simulink model "simRouteA_v4_11"  (R2015a)
settings: Solver=FixedStepDiscrete  StartTime=0.0  StopTime=36000  FixedStep=1  RelTol=1e-3
PreLoadFcn:
  | loadTimetable
StopFcn:
  | postProcess
undefined symbols (not defined in the file or in its folder): setBus1IntergenTime, setBus2IntergenTime, setBus3IntergenTime, setBus4IntergenTime
(part 5 of 7)

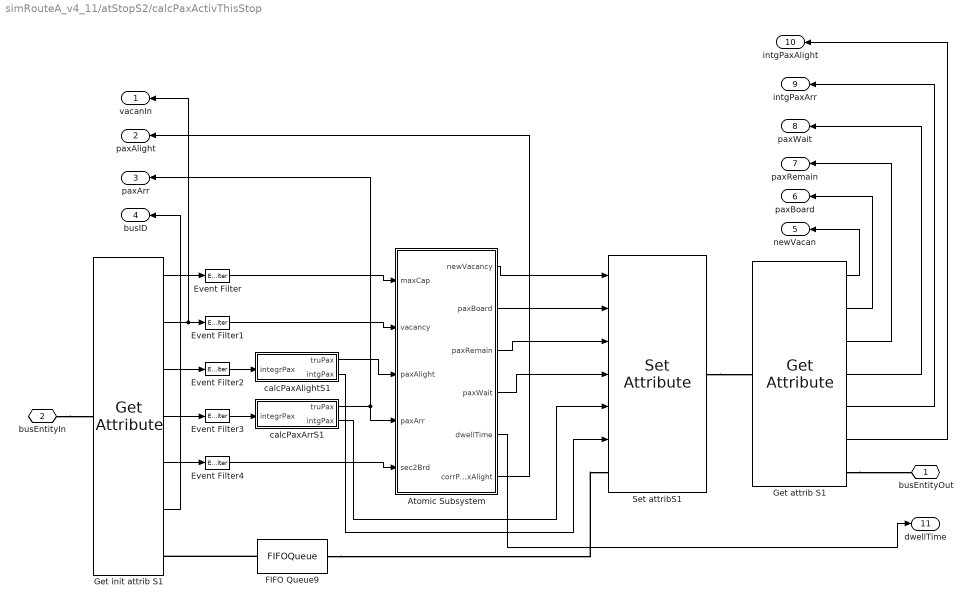
== system simRouteA_v4_11/atStopS2/calcPaxActivThisStop ==
  Atomic Subsystem : Subsystem  TreatAsAtomicUnit=on
  Event Filter{,1..4} (5 alike) : EventFilter  ExecuteSubsystem=Upon sample time hit  SignalEdgeType=Rising
  FIFO Queue9 : FIFOQueue
  Get attrib S1 : GetAttribute  AttributeName=vacancy|paxBoard|paxRemain|paxWait|intgPaxArr|intgPaxAlight  AttributeMissing=Error|Error|Error|Error|Error|Error  AttributeDefaultValue=1|1|1|1|1|1  AttributeTreatAsVector=1|1|1|1|1|1  AttributeSendTiming=After entity departure|After entity departure|After entity departure|After entity departure|After entity departure|After entity departure  EvaluatedDefaultAttributeValue={ []; []; []; []; []; []}
      settings: OutputPortMap=o1,o2,o3,o4,o5,o6
  Get init attrib S1 : GetAttribute  AttributeName=maxCap|vacancy|paxAlight|paxArr|sec2Brd|ID  AttributeMissing=Error|Error|Error|Error|Error|Error  AttributeDefaultValue=1|1|1|1|1|1  AttributeTreatAsVector=1|1|1|1|1|1  AttributeSendTiming=After entity departure|After entity departure|After entity departure|After entity departure|After entity departure|After entity departure  EvaluatedDefaultAttributeValue={ []; []; []; []; []; []}
      settings: OutputPortMap=o1,o2,o3,o4,o5,o6
  Set attribS1 : SetAttribute  AttributeName=vacancy|paxBoard|paxRemain|paxWait|intgPaxArr|intgPaxAlight  AttributeFrom=Signal port|Signal port|Signal port|Signal port|Signal port|Signal port  AttributeValue=1|1|1|1|1|1  AttributeTreatAsVector=1|1|1|1|1|1  EvaluatedAttributeValue={ []; []; []; []; []; [] }
      settings: InputPortMap=u0,u1,u2,u3,u4,u5
  calcPaxAlightS1 : Subsystem  TreatAsAtomicUnit=on
  calcPaxArrS1 : Subsystem  TreatAsAtomicUnit=on
  busEntityOut : PMIOPort  Port=1  Side=Right
  busEntityIn : PMIOPort  Port=2  Side=Left
  vacanIn : Outport
  paxAlight : Outport  Port=2
  paxArr : Outport  Port=3
  busID : Outport  Port=4
  newVacan : Outport  Port=5
  paxBoard : Outport  Port=6
  paxRemain : Outport  Port=7
  paxWait : Outport  Port=8
  intgPaxArr : Outport  Port=9
  intgPaxAlight : Outport  Port=10
  dwellTime : Outport  Port=11
  wires:
  Event Filter3/1 -> calcPaxArrS1/1(integrPax)
  Event Filter2/1 -> calcPaxAlightS1/1(integrPax)
  Get init attrib S1/6 -> busID/1
  Get init attrib S1/2 -> vacanIn/1, Event Filter1/1
  Get attrib S1/2 -> paxBoard/1
  Atomic Subsystem/1(newVacancy) -> Set attribS1/1
  Get attrib S1/1 -> newVacan/1
  Get attrib S1/3 -> paxRemain/1
  Get attrib S1/4 -> paxWait/1
  Event Filter/1 -> Atomic Subsystem/1(maxCap)
  Get init attrib S1/5 -> Event Filter4/1
  Atomic Subsystem/5(dwellTime) -> dwellTime/1
  Event Filter1/1 -> Atomic Subsystem/2(vacancy)
  Get init attrib S1/1 -> Event Filter/1
  Event Filter4/1 -> Atomic Subsystem/5(sec2Brd)
  Atomic Subsystem/2(paxBoard) -> Set attribS1/2
  Atomic Subsystem/3(paxRemain) -> Set attribS1/3
  Atomic Subsystem/4(paxWait) -> Set attribS1/4
  Get init attrib S1/4 -> Event Filter3/1
  Get init attrib S1/3 -> Event Filter2/1
  calcPaxAlightS1/1(truPax) -> Atomic Subsystem/3(paxAlight)
  calcPaxArrS1/1(truPax) -> Atomic Subsystem/4(paxArr), paxArr/1
  calcPaxArrS1/2(intgPax) -> Set attribS1/5
  calcPaxAlightS1/2(intgPax) -> Set attribS1/6
  Get attrib S1/5 -> intgPaxArr/1
  Get attrib S1/6 -> intgPaxAlight/1
  Atomic Subsystem/6(corrPaxAlight) -> paxAlight/1
  connections:
  busEntityIn/RConn1 -- Get init attrib S1/LConn1
  FIFO Queue9/LConn1 -- Get init attrib S1/RConn1
  Set attribS1/RConn1 -- Get attrib S1/LConn1
  Get attrib S1/RConn1 -- busEntityOut/RConn1
  FIFO Queue9/RConn1 -- Set attribS1/LConn1

== system simRouteA_v4_11/atStopS2/integrPaxAlightS1 ==
  ratePax : Inport
  Atomic Subsystem1 : Subsystem  TreatAsAtomicUnit=on
  Round1 : Rounding  Operator=round
  T2E1 : TimedToEventSignal
  accPax : Outport
  wires:
  Round1/1 -> T2E1/1
  T2E1/1 -> Atomic Subsystem1/1(In1)
  ratePax/1 -> Round1/1
  Atomic Subsystem1/1(Out1) -> accPax/1

== system simRouteA_v4_11/atStopS2/integrPaxArrS1 ==
  ratePax : Inport
  Atomic Subsystem1 : Subsystem  TreatAsAtomicUnit=on
  Round1 : Rounding  Operator=round
  T2E1 : TimedToEventSignal
  accPax : Outport
  wires:
  Round1/1 -> T2E1/1
  T2E1/1 -> Atomic Subsystem1/1(In1)
  ratePax/1 -> Round1/1
  Atomic Subsystem1/1(Out1) -> accPax/1

== system simRouteA_v4_11/atStopS3/busDwellThisStop ==
  dwellTime : Inport
  Clock2 : Clock
  DummyServer : SingleServer  ServiceTime=0
  FIFO Queue3 : FIFOQueue
  Get Attribute5 : GetAttribute  AttributeName=dwellTime|tStartSrvPax  AttributeMissing=Error|Error  AttributeDefaultValue=1|1  AttributeTreatAsVector=1|1  AttributeSendTiming=After entity departure|After entity departure  EvaluatedDefaultAttributeValue={ []; []}
      settings: OutputPortMap=o1,o2
  Infinite Server : InfiniteServer  ServiceTimeFrom=Signal port t
  Set Attribute3 : SetAttribute  AttributeName=dwellTime|tStartSrvPax  AttributeFrom=Signal port|Signal port  AttributeValue=1|1  AttributeTreatAsVector=1|1  EvaluatedAttributeValue={ []; [] }
      settings: InputPortMap=u0,u1
  Subsystem2 : Subsystem  TreatAsAtomicUnit=on
  T2E4 : TimedToEventSignal
  busWaitAtStop : SingleServer  Commented=on  ServiceTimeFrom=Signal port t
  busesQueueAtStop : FIFOQueue
  getIDBusLeave : GetAttribute  AttributeName=ID  EvaluatedDefaultAttributeValue={ []}
      settings: OutputPortMap=o1
  busOut : PMIOPort  Port=1  Side=Right
  busIn : PMIOPort  Port=2  Side=Left
  idBusLeave : Outport
  wires:
  getIDBusLeave/1 -> idBusLeave/1
  dwellTime/1 -> Set Attribute3/1
  Clock2/1 -> T2E4/1
  T2E4/1 -> Set Attribute3/2
  Get Attribute5/2 -> Subsystem2/2(tStartSrvPax)
  Get Attribute5/1 -> Subsystem2/1(dwellTime)
  Subsystem2/1(dwellTimeNew) -> Infinite Server/1
  connections:
  busIn/RConn1 -- busesQueueAtStop/LConn1
  getIDBusLeave/RConn1 -- busOut/RConn1
  busesQueueAtStop/RConn1 -- Set Attribute3/LConn1
  Infinite Server/RConn1 -- getIDBusLeave/LConn1
  Set Attribute3/RConn1 -- FIFO Queue3/LConn1
  FIFO Queue3/RConn1 -- Get Attribute5/LConn1
  Get Attribute5/RConn1 -- DummyServer/LConn1
  Infinite Server/LConn1 -- DummyServer/RConn1

== system simRouteA_v4_11/atStopS3/calcPaxActivThisStop ==
  Atomic Subsystem : Subsystem  TreatAsAtomicUnit=on
  Event Filter{,1..4} (5 alike) : EventFilter  ExecuteSubsystem=Upon sample time hit  SignalEdgeType=Rising
  FIFO Queue9 : FIFOQueue
  Get attrib S1 : GetAttribute  AttributeName=vacancy|paxBoard|paxRemain|paxWait|intgPaxArr|intgPaxAlight  AttributeMissing=Error|Error|Error|Error|Error|Error  AttributeDefaultValue=1|1|1|1|1|1  AttributeTreatAsVector=1|1|1|1|1|1  AttributeSendTiming=After entity departure|After entity departure|After entity departure|After entity departure|After entity departure|After entity departure  EvaluatedDefaultAttributeValue={ []; []; []; []; []; []}
      settings: OutputPortMap=o1,o2,o3,o4,o5,o6
  Get init attrib S1 : GetAttribute  AttributeName=maxCap|vacancy|paxAlight|paxArr|sec2Brd|ID  AttributeMissing=Error|Error|Error|Error|Error|Error  AttributeDefaultValue=1|1|1|1|1|1  AttributeTreatAsVector=1|1|1|1|1|1  AttributeSendTiming=After entity departure|After entity departure|After entity departure|After entity departure|After entity departure|After entity departure  EvaluatedDefaultAttributeValue={ []; []; []; []; []; []}
      settings: OutputPortMap=o1,o2,o3,o4,o5,o6
  Set attribS1 : SetAttribute  AttributeName=vacancy|paxBoard|paxRemain|paxWait|intgPaxArr|intgPaxAlight  AttributeFrom=Signal port|Signal port|Signal port|Signal port|Signal port|Signal port  AttributeValue=1|1|1|1|1|1  AttributeTreatAsVector=1|1|1|1|1|1  EvaluatedAttributeValue={ []; []; []; []; []; [] }
      settings: InputPortMap=u0,u1,u2,u3,u4,u5
  calcPaxAlightS1 : Subsystem  TreatAsAtomicUnit=on
  calcPaxArrS1 : Subsystem  TreatAsAtomicUnit=on
  busEntityOut : PMIOPort  Port=1  Side=Right
  busEntityIn : PMIOPort  Port=2  Side=Left
  vacanIn : Outport
  paxAlight : Outport  Port=2
  paxArr : Outport  Port=3
  busID : Outport  Port=4
  newVacan : Outport  Port=5
  paxBoard : Outport  Port=6
  paxRemain : Outport  Port=7
  paxWait : Outport  Port=8
  intgPaxArr : Outport  Port=9
  intgPaxAlight : Outport  Port=10
  dwellTime : Outport  Port=11
  wires:
  Event Filter3/1 -> calcPaxArrS1/1(integrPax)
  Event Filter2/1 -> calcPaxAlightS1/1(integrPax)
  Get init attrib S1/6 -> busID/1
  Get init attrib S1/2 -> vacanIn/1, Event Filter1/1
  Get attrib S1/2 -> paxBoard/1
  Atomic Subsystem/1(newVacancy) -> Set attribS1/1
  Get attrib S1/1 -> newVacan/1
  Get attrib S1/3 -> paxRemain/1
  Get attrib S1/4 -> paxWait/1
  Event Filter/1 -> Atomic Subsystem/1(maxCap)
  Get init attrib S1/5 -> Event Filter4/1
  Atomic Subsystem/5(dwellTime) -> dwellTime/1
  Event Filter1/1 -> Atomic Subsystem/2(vacancy)
  Get init attrib S1/1 -> Event Filter/1
  Event Filter4/1 -> Atomic Subsystem/5(sec2Brd)
  Atomic Subsystem/2(paxBoard) -> Set attribS1/2
  Atomic Subsystem/3(paxRemain) -> Set attribS1/3
  Atomic Subsystem/4(paxWait) -> Set attribS1/4
  Get init attrib S1/4 -> Event Filter3/1
  Get init attrib S1/3 -> Event Filter2/1
  calcPaxAlightS1/1(truPax) -> Atomic Subsystem/3(paxAlight)
  calcPaxArrS1/1(truPax) -> Atomic Subsystem/4(paxArr), paxArr/1
  calcPaxArrS1/2(intgPax) -> Set attribS1/5
  calcPaxAlightS1/2(intgPax) -> Set attribS1/6
  Get attrib S1/5 -> intgPaxArr/1
  Get attrib S1/6 -> intgPaxAlight/1
  Atomic Subsystem/6(corrPaxAlight) -> paxAlight/1
  connections:
  busEntityIn/RConn1 -- Get init attrib S1/LConn1
  FIFO Queue9/LConn1 -- Get init attrib S1/RConn1
  Set attribS1/RConn1 -- Get attrib S1/LConn1
  Get attrib S1/RConn1 -- busEntityOut/RConn1
  FIFO Queue9/RConn1 -- Set attribS1/LConn1

== system simRouteA_v4_11/atStopS3/integrPaxAlightS1 ==
  ratePax : Inport
  Atomic Subsystem1 : Subsystem  TreatAsAtomicUnit=on
  Round1 : Rounding  Operator=round
  T2E1 : TimedToEventSignal
  accPax : Outport
  wires:
  Round1/1 -> T2E1/1
  T2E1/1 -> Atomic Subsystem1/1(In1)
  ratePax/1 -> Round1/1
  Atomic Subsystem1/1(Out1) -> accPax/1

== system simRouteA_v4_11/atStopS3/integrPaxArrS1 ==
  ratePax : Inport
  Atomic Subsystem1 : Subsystem  TreatAsAtomicUnit=on
  Round1 : Rounding  Operator=round
  T2E1 : TimedToEventSignal
  accPax : Outport
  wires:
  Round1/1 -> T2E1/1
  T2E1/1 -> Atomic Subsystem1/1(In1)
  ratePax/1 -> Round1/1
  Atomic Subsystem1/1(Out1) -> accPax/1

== system simRouteA_v4_11/atStopS4/busDwellThisStop ==
  dwellTime : Inport
  Clock2 : Clock
  DummyServer : SingleServer  ServiceTime=0
  FIFO Queue3 : FIFOQueue
  Get Attribute5 : GetAttribute  AttributeName=dwellTime|tStartSrvPax  AttributeMissing=Error|Error  AttributeDefaultValue=1|1  AttributeTreatAsVector=1|1  AttributeSendTiming=After entity departure|After entity departure  EvaluatedDefaultAttributeValue={ []; []}
      settings: OutputPortMap=o1,o2
  Infinite Server : InfiniteServer  ServiceTimeFrom=Signal port t
  Set Attribute3 : SetAttribute  AttributeName=dwellTime|tStartSrvPax  AttributeFrom=Signal port|Signal port  AttributeValue=1|1  AttributeTreatAsVector=1|1  EvaluatedAttributeValue={ []; [] }
      settings: InputPortMap=u0,u1
  Subsystem2 : Subsystem  TreatAsAtomicUnit=on
  T2E4 : TimedToEventSignal
  busWaitAtStop : SingleServer  Commented=on  ServiceTimeFrom=Signal port t
  busesQueueAtStop : FIFOQueue
  getIDBusLeave : GetAttribute  AttributeName=ID  EvaluatedDefaultAttributeValue={ []}
      settings: OutputPortMap=o1
  busOut : PMIOPort  Port=1  Side=Right
  busIn : PMIOPort  Port=2  Side=Left
  idBusLeave : Outport
  wires:
  getIDBusLeave/1 -> idBusLeave/1
  dwellTime/1 -> Set Attribute3/1
  Clock2/1 -> T2E4/1
  T2E4/1 -> Set Attribute3/2
  Get Attribute5/2 -> Subsystem2/2(tStartSrvPax)
  Get Attribute5/1 -> Subsystem2/1(dwellTime)
  Subsystem2/1(dwellTimeNew) -> Infinite Server/1
  connections:
  busIn/RConn1 -- busesQueueAtStop/LConn1
  getIDBusLeave/RConn1 -- busOut/RConn1
  busesQueueAtStop/RConn1 -- Set Attribute3/LConn1
  Infinite Server/RConn1 -- getIDBusLeave/LConn1
  Set Attribute3/RConn1 -- FIFO Queue3/LConn1
  FIFO Queue3/RConn1 -- Get Attribute5/LConn1
  Get Attribute5/RConn1 -- DummyServer/LConn1
  Infinite Server/LConn1 -- DummyServer/RConn1

== system simRouteA_v4_11/atStopS4/calcPaxActivThisStop ==
  Atomic Subsystem : Subsystem  TreatAsAtomicUnit=on
  Event Filter{,1..4} (5 alike) : EventFilter  ExecuteSubsystem=Upon sample time hit  SignalEdgeType=Rising
  FIFO Queue9 : FIFOQueue
  Get attrib S1 : GetAttribute  AttributeName=vacancy|paxBoard|paxRemain|paxWait|intgPaxArr|intgPaxAlight  AttributeMissing=Error|Error|Error|Error|Error|Error  AttributeDefaultValue=1|1|1|1|1|1  AttributeTreatAsVector=1|1|1|1|1|1  AttributeSendTiming=After entity departure|After entity departure|After entity departure|After entity departure|After entity departure|After entity departure  EvaluatedDefaultAttributeValue={ []; []; []; []; []; []}
      settings: OutputPortMap=o1,o2,o3,o4,o5,o6
  Get init attrib S1 : GetAttribute  AttributeName=maxCap|vacancy|paxAlight|paxArr|sec2Brd|ID  AttributeMissing=Error|Error|Error|Error|Error|Error  AttributeDefaultValue=1|1|1|1|1|1  AttributeTreatAsVector=1|1|1|1|1|1  AttributeSendTiming=After entity departure|After entity departure|After entity departure|After entity departure|After entity departure|After entity departure  EvaluatedDefaultAttributeValue={ []; []; []; []; []; []}
      settings: OutputPortMap=o1,o2,o3,o4,o5,o6
  Set attribS1 : SetAttribute  AttributeName=vacancy|paxBoard|paxRemain|paxWait|intgPaxArr|intgPaxAlight  AttributeFrom=Signal port|Signal port|Signal port|Signal port|Signal port|Signal port  AttributeValue=1|1|1|1|1|1  AttributeTreatAsVector=1|1|1|1|1|1  EvaluatedAttributeValue={ []; []; []; []; []; [] }
      settings: InputPortMap=u0,u1,u2,u3,u4,u5
  calcPaxAlightS1 : Subsystem  TreatAsAtomicUnit=on
  calcPaxArrS1 : Subsystem  TreatAsAtomicUnit=on
  busEntityOut : PMIOPort  Port=1  Side=Right
  busEntityIn : PMIOPort  Port=2  Side=Left
  vacanIn : Outport
  paxAlight : Outport  Port=2
  paxArr : Outport  Port=3
  busID : Outport  Port=4
  newVacan : Outport  Port=5
  paxBoard : Outport  Port=6
  paxRemain : Outport  Port=7
  paxWait : Outport  Port=8
  intgPaxArr : Outport  Port=9
  intgPaxAlight : Outport  Port=10
  dwellTime : Outport  Port=11
  wires:
  Event Filter3/1 -> calcPaxArrS1/1(integrPax)
  Event Filter2/1 -> calcPaxAlightS1/1(integrPax)
  Get init attrib S1/6 -> busID/1
  Get init attrib S1/2 -> vacanIn/1, Event Filter1/1
  Get attrib S1/2 -> paxBoard/1
  Atomic Subsystem/1(newVacancy) -> Set attribS1/1
  Get attrib S1/1 -> newVacan/1
  Get attrib S1/3 -> paxRemain/1
  Get attrib S1/4 -> paxWait/1
  Event Filter/1 -> Atomic Subsystem/1(maxCap)
  Get init attrib S1/5 -> Event Filter4/1
  Atomic Subsystem/5(dwellTime) -> dwellTime/1
  Event Filter1/1 -> Atomic Subsystem/2(vacancy)
  Get init attrib S1/1 -> Event Filter/1
  Event Filter4/1 -> Atomic Subsystem/5(sec2Brd)
  Atomic Subsystem/2(paxBoard) -> Set attribS1/2
  Atomic Subsystem/3(paxRemain) -> Set attribS1/3
  Atomic Subsystem/4(paxWait) -> Set attribS1/4
  Get init attrib S1/4 -> Event Filter3/1
  Get init attrib S1/3 -> Event Filter2/1
  calcPaxAlightS1/1(truPax) -> Atomic Subsystem/3(paxAlight)
  calcPaxArrS1/1(truPax) -> Atomic Subsystem/4(paxArr), paxArr/1
  calcPaxArrS1/2(intgPax) -> Set attribS1/5
  calcPaxAlightS1/2(intgPax) -> Set attribS1/6
  Get attrib S1/5 -> intgPaxArr/1
  Get attrib S1/6 -> intgPaxAlight/1
  Atomic Subsystem/6(corrPaxAlight) -> paxAlight/1
  connections:
  busEntityIn/RConn1 -- Get init attrib S1/LConn1
  FIFO Queue9/LConn1 -- Get init attrib S1/RConn1
  Set attribS1/RConn1 -- Get attrib S1/LConn1
  Get attrib S1/RConn1 -- busEntityOut/RConn1
  FIFO Queue9/RConn1 -- Set attribS1/LConn1

== system simRouteA_v4_11/atStopS4/integrPaxAlightS1 ==
  ratePax : Inport
  Atomic Subsystem1 : Subsystem  TreatAsAtomicUnit=on
  Round1 : Rounding  Operator=round
  T2E1 : TimedToEventSignal
  accPax : Outport
  wires:
  Round1/1 -> T2E1/1
  T2E1/1 -> Atomic Subsystem1/1(In1)
  ratePax/1 -> Round1/1
  Atomic Subsystem1/1(Out1) -> accPax/1

== system simRouteA_v4_11/atStopS4/integrPaxArrS1 ==
  ratePax : Inport
  Atomic Subsystem1 : Subsystem  TreatAsAtomicUnit=on
  Round1 : Rounding  Operator=round
  T2E1 : TimedToEventSignal
  accPax : Outport
  wires:
  Round1/1 -> T2E1/1
  T2E1/1 -> Atomic Subsystem1/1(In1)
  ratePax/1 -> Round1/1
  Atomic Subsystem1/1(Out1) -> accPax/1

== system simRouteA_v4_11/atStopS5/busDwellThisStop ==
  dwellTime : Inport
  Clock2 : Clock
  DummyServer : SingleServer  ServiceTime=0
  FIFO Queue3 : FIFOQueue
  Get Attribute5 : GetAttribute  AttributeName=dwellTime|tStartSrvPax  AttributeMissing=Error|Error  AttributeDefaultValue=1|1  AttributeTreatAsVector=1|1  AttributeSendTiming=After entity departure|After entity departure  EvaluatedDefaultAttributeValue={ []; []}
      settings: OutputPortMap=o1,o2
  Infinite Server : InfiniteServer  ServiceTimeFrom=Signal port t
  Set Attribute3 : SetAttribute  AttributeName=dwellTime|tStartSrvPax  AttributeFrom=Signal port|Signal port  AttributeValue=1|1  AttributeTreatAsVector=1|1  EvaluatedAttributeValue={ []; [] }
      settings: InputPortMap=u0,u1
  Subsystem2 : Subsystem  TreatAsAtomicUnit=on
  T2E4 : TimedToEventSignal
  busWaitAtStop : SingleServer  Commented=on  ServiceTimeFrom=Signal port t
  busesQueueAtStop : FIFOQueue
  getIDBusLeave : GetAttribute  AttributeName=ID  EvaluatedDefaultAttributeValue={ []}
      settings: OutputPortMap=o1
  busOut : PMIOPort  Port=1  Side=Right
  busIn : PMIOPort  Port=2  Side=Left
  idBusLeave : Outport
  wires:
  getIDBusLeave/1 -> idBusLeave/1
  dwellTime/1 -> Set Attribute3/1
  Clock2/1 -> T2E4/1
  T2E4/1 -> Set Attribute3/2
  Get Attribute5/2 -> Subsystem2/2(tStartSrvPax)
  Get Attribute5/1 -> Subsystem2/1(dwellTime)
  Subsystem2/1(dwellTimeNew) -> Infinite Server/1
  connections:
  busIn/RConn1 -- busesQueueAtStop/LConn1
  getIDBusLeave/RConn1 -- busOut/RConn1
  busesQueueAtStop/RConn1 -- Set Attribute3/LConn1
  Infinite Server/RConn1 -- getIDBusLeave/LConn1
  Set Attribute3/RConn1 -- FIFO Queue3/LConn1
  FIFO Queue3/RConn1 -- Get Attribute5/LConn1
  Get Attribute5/RConn1 -- DummyServer/LConn1
  Infinite Server/LConn1 -- DummyServer/RConn1

== system simRouteA_v4_11/atStopS5/calcPaxActivThisStop ==
  Atomic Subsystem : Subsystem  TreatAsAtomicUnit=on
  Event Filter{,1..4} (5 alike) : EventFilter  ExecuteSubsystem=Upon sample time hit  SignalEdgeType=Rising
  FIFO Queue9 : FIFOQueue
  Get attrib S1 : GetAttribute  AttributeName=vacancy|paxBoard|paxRemain|paxWait|intgPaxArr|intgPaxAlight  AttributeMissing=Error|Error|Error|Error|Error|Error  AttributeDefaultValue=1|1|1|1|1|1  AttributeTreatAsVector=1|1|1|1|1|1  AttributeSendTiming=After entity departure|After entity departure|After entity departure|After entity departure|After entity departure|After entity departure  EvaluatedDefaultAttributeValue={ []; []; []; []; []; []}
      settings: OutputPortMap=o1,o2,o3,o4,o5,o6
  Get init attrib S1 : GetAttribute  AttributeName=maxCap|vacancy|paxAlight|paxArr|sec2Brd|ID  AttributeMissing=Error|Error|Error|Error|Error|Error  AttributeDefaultValue=1|1|1|1|1|1  AttributeTreatAsVector=1|1|1|1|1|1  AttributeSendTiming=After entity departure|After entity departure|After entity departure|After entity departure|After entity departure|After entity departure  EvaluatedDefaultAttributeValue={ []; []; []; []; []; []}
      settings: OutputPortMap=o1,o2,o3,o4,o5,o6
  Set attribS1 : SetAttribute  AttributeName=vacancy|paxBoard|paxRemain|paxWait|intgPaxArr|intgPaxAlight  AttributeFrom=Signal port|Signal port|Signal port|Signal port|Signal port|Signal port  AttributeValue=1|1|1|1|1|1  AttributeTreatAsVector=1|1|1|1|1|1  EvaluatedAttributeValue={ []; []; []; []; []; [] }
      settings: InputPortMap=u0,u1,u2,u3,u4,u5
  calcPaxAlightS1 : Subsystem  TreatAsAtomicUnit=on
  calcPaxArrS1 : Subsystem  TreatAsAtomicUnit=on
  busEntityOut : PMIOPort  Port=1  Side=Right
  busEntityIn : PMIOPort  Port=2  Side=Left
  vacanIn : Outport
  paxAlight : Outport  Port=2
  paxArr : Outport  Port=3
  busID : Outport  Port=4
  newVacan : Outport  Port=5
  paxBoard : Outport  Port=6
  paxRemain : Outport  Port=7
  paxWait : Outport  Port=8
  intgPaxArr : Outport  Port=9
  intgPaxAlight : Outport  Port=10
  dwellTime : Outport  Port=11
  wires:
  Event Filter3/1 -> calcPaxArrS1/1(integrPax)
  Event Filter2/1 -> calcPaxAlightS1/1(integrPax)
  Get init attrib S1/6 -> busID/1
  Get init attrib S1/2 -> vacanIn/1, Event Filter1/1
  Get attrib S1/2 -> paxBoard/1
  Atomic Subsystem/1(newVacancy) -> Set attribS1/1
  Get attrib S1/1 -> newVacan/1
  Get attrib S1/3 -> paxRemain/1
  Get attrib S1/4 -> paxWait/1
  Event Filter/1 -> Atomic Subsystem/1(maxCap)
  Get init attrib S1/5 -> Event Filter4/1
  Atomic Subsystem/5(dwellTime) -> dwellTime/1
  Event Filter1/1 -> Atomic Subsystem/2(vacancy)
  Get init attrib S1/1 -> Event Filter/1
  Event Filter4/1 -> Atomic Subsystem/5(sec2Brd)
  Atomic Subsystem/2(paxBoard) -> Set attribS1/2
  Atomic Subsystem/3(paxRemain) -> Set attribS1/3
  Atomic Subsystem/4(paxWait) -> Set attribS1/4
  Get init attrib S1/4 -> Event Filter3/1
  Get init attrib S1/3 -> Event Filter2/1
  calcPaxAlightS1/1(truPax) -> Atomic Subsystem/3(paxAlight)
  calcPaxArrS1/1(truPax) -> Atomic Subsystem/4(paxArr), paxArr/1
  calcPaxArrS1/2(intgPax) -> Set attribS1/5
  calcPaxAlightS1/2(intgPax) -> Set attribS1/6
  Get attrib S1/5 -> intgPaxArr/1
  Get attrib S1/6 -> intgPaxAlight/1
  Atomic Subsystem/6(corrPaxAlight) -> paxAlight/1
  connections:
  busEntityIn/RConn1 -- Get init attrib S1/LConn1
  FIFO Queue9/LConn1 -- Get init attrib S1/RConn1
  Set attribS1/RConn1 -- Get attrib S1/LConn1
  Get attrib S1/RConn1 -- busEntityOut/RConn1
  FIFO Queue9/RConn1 -- Set attribS1/LConn1

== system simRouteA_v4_11/atStopS5/integrPaxAlightS1 ==
  ratePax : Inport
  Atomic Subsystem1 : Subsystem  TreatAsAtomicUnit=on
  Round1 : Rounding  Operator=round
  T2E1 : TimedToEventSignal
  accPax : Outport
  wires:
  Round1/1 -> T2E1/1
  T2E1/1 -> Atomic Subsystem1/1(In1)
  ratePax/1 -> Round1/1
  Atomic Subsystem1/1(Out1) -> accPax/1

== system simRouteA_v4_11/atStopS5/integrPaxArrS1 ==
  ratePax : Inport
  Atomic Subsystem1 : Subsystem  TreatAsAtomicUnit=on
  Round1 : Rounding  Operator=round
  T2E1 : TimedToEventSignal
  accPax : Outport
  wires:
  Round1/1 -> T2E1/1
  T2E1/1 -> Atomic Subsystem1/1(In1)
  ratePax/1 -> Round1/1
  Atomic Subsystem1/1(Out1) -> accPax/1

== system simRouteA_v4_11/atStopS6/busDwellThisStop ==
  dwellTime : Inport
  Clock2 : Clock
  DummyServer : SingleServer  ServiceTime=0
  FIFO Queue3 : FIFOQueue
  Get Attribute5 : GetAttribute  AttributeName=dwellTime|tStartSrvPax  AttributeMissing=Error|Error  AttributeDefaultValue=1|1  AttributeTreatAsVector=1|1  AttributeSendTiming=After entity departure|After entity departure  EvaluatedDefaultAttributeValue={ []; []}
      settings: OutputPortMap=o1,o2
  Infinite Server : InfiniteServer  ServiceTimeFrom=Signal port t
  Set Attribute3 : SetAttribute  AttributeName=dwellTime|tStartSrvPax  AttributeFrom=Signal port|Signal port  AttributeValue=1|1  AttributeTreatAsVector=1|1  EvaluatedAttributeValue={ []; [] }
      settings: InputPortMap=u0,u1
  Subsystem2 : Subsystem  TreatAsAtomicUnit=on
  T2E4 : TimedToEventSignal
  busWaitAtStop : SingleServer  Commented=on  ServiceTimeFrom=Signal port t
  busesQueueAtStop : FIFOQueue
  getIDBusLeave : GetAttribute  AttributeName=ID  EvaluatedDefaultAttributeValue={ []}
      settings: OutputPortMap=o1
  busOut : PMIOPort  Port=1  Side=Right
  busIn : PMIOPort  Port=2  Side=Left
  idBusLeave : Outport
  wires:
  getIDBusLeave/1 -> idBusLeave/1
  dwellTime/1 -> Set Attribute3/1
  Clock2/1 -> T2E4/1
  T2E4/1 -> Set Attribute3/2
  Get Attribute5/2 -> Subsystem2/2(tStartSrvPax)
  Get Attribute5/1 -> Subsystem2/1(dwellTime)
  Subsystem2/1(dwellTimeNew) -> Infinite Server/1
  connections:
  busIn/RConn1 -- busesQueueAtStop/LConn1
  getIDBusLeave/RConn1 -- busOut/RConn1
  busesQueueAtStop/RConn1 -- Set Attribute3/LConn1
  Infinite Server/RConn1 -- getIDBusLeave/LConn1
  Set Attribute3/RConn1 -- FIFO Queue3/LConn1
  FIFO Queue3/RConn1 -- Get Attribute5/LConn1
  Get Attribute5/RConn1 -- DummyServer/LConn1
  Infinite Server/LConn1 -- DummyServer/RConn1

== system simRouteA_v4_11/atStopS6/calcPaxActivThisStop ==
  Atomic Subsystem : Subsystem  TreatAsAtomicUnit=on
  Event Filter{,1..4} (5 alike) : EventFilter  ExecuteSubsystem=Upon sample time hit  SignalEdgeType=Rising
  FIFO Queue9 : FIFOQueue
  Get attrib S1 : GetAttribute  AttributeName=vacancy|paxBoard|paxRemain|paxWait|intgPaxArr|intgPaxAlight  AttributeMissing=Error|Error|Error|Error|Error|Error  AttributeDefaultValue=1|1|1|1|1|1  AttributeTreatAsVector=1|1|1|1|1|1  AttributeSendTiming=After entity departure|After entity departure|After entity departure|After entity departure|After entity departure|After entity departure  EvaluatedDefaultAttributeValue={ []; []; []; []; []; []}
      settings: OutputPortMap=o1,o2,o3,o4,o5,o6
  Get init attrib S1 : GetAttribute  AttributeName=maxCap|vacancy|paxAlight|paxArr|sec2Brd|ID  AttributeMissing=Error|Error|Error|Error|Error|Error  AttributeDefaultValue=1|1|1|1|1|1  AttributeTreatAsVector=1|1|1|1|1|1  AttributeSendTiming=After entity departure|After entity departure|After entity departure|After entity departure|After entity departure|After entity departure  EvaluatedDefaultAttributeValue={ []; []; []; []; []; []}
      settings: OutputPortMap=o1,o2,o3,o4,o5,o6
  Set attribS1 : SetAttribute  AttributeName=vacancy|paxBoard|paxRemain|paxWait|intgPaxArr|intgPaxAlight  AttributeFrom=Signal port|Signal port|Signal port|Signal port|Signal port|Signal port  AttributeValue=1|1|1|1|1|1  AttributeTreatAsVector=1|1|1|1|1|1  EvaluatedAttributeValue={ []; []; []; []; []; [] }
      settings: InputPortMap=u0,u1,u2,u3,u4,u5
  calcPaxAlightS1 : Subsystem  TreatAsAtomicUnit=on
  calcPaxArrS1 : Subsystem  TreatAsAtomicUnit=on
  busEntityOut : PMIOPort  Port=1  Side=Right
  busEntityIn : PMIOPort  Port=2  Side=Left
  vacanIn : Outport
  paxAlight : Outport  Port=2
  paxArr : Outport  Port=3
  busID : Outport  Port=4
  newVacan : Outport  Port=5
  paxBoard : Outport  Port=6
  paxRemain : Outport  Port=7
  paxWait : Outport  Port=8
  intgPaxArr : Outport  Port=9
  intgPaxAlight : Outport  Port=10
  dwellTime : Outport  Port=11
  wires:
  Event Filter3/1 -> calcPaxArrS1/1(integrPax)
  Event Filter2/1 -> calcPaxAlightS1/1(integrPax)
  Get init attrib S1/6 -> busID/1
  Get init attrib S1/2 -> vacanIn/1, Event Filter1/1
  Get attrib S1/2 -> paxBoard/1
  Atomic Subsystem/1(newVacancy) -> Set attribS1/1
  Get attrib S1/1 -> newVacan/1
  Get attrib S1/3 -> paxRemain/1
  Get attrib S1/4 -> paxWait/1
  Event Filter/1 -> Atomic Subsystem/1(maxCap)
  Get init attrib S1/5 -> Event Filter4/1
  Atomic Subsystem/5(dwellTime) -> dwellTime/1
  Event Filter1/1 -> Atomic Subsystem/2(vacancy)
  Get init attrib S1/1 -> Event Filter/1
  Event Filter4/1 -> Atomic Subsystem/5(sec2Brd)
  Atomic Subsystem/2(paxBoard) -> Set attribS1/2
  Atomic Subsystem/3(paxRemain) -> Set attribS1/3
  Atomic Subsystem/4(paxWait) -> Set attribS1/4
  Get init attrib S1/4 -> Event Filter3/1
  Get init attrib S1/3 -> Event Filter2/1
  calcPaxAlightS1/1(truPax) -> Atomic Subsystem/3(paxAlight)
  calcPaxArrS1/1(truPax) -> Atomic Subsystem/4(paxArr), paxArr/1
  calcPaxArrS1/2(intgPax) -> Set attribS1/5
  calcPaxAlightS1/2(intgPax) -> Set attribS1/6
  Get attrib S1/5 -> intgPaxArr/1
  Get attrib S1/6 -> intgPaxAlight/1
  Atomic Subsystem/6(corrPaxAlight) -> paxAlight/1
  connections:
  busEntityIn/RConn1 -- Get init attrib S1/LConn1
  FIFO Queue9/LConn1 -- Get init attrib S1/RConn1
  Set attribS1/RConn1 -- Get attrib S1/LConn1
  Get attrib S1/RConn1 -- busEntityOut/RConn1
  FIFO Queue9/RConn1 -- Set attribS1/LConn1

== system simRouteA_v4_11/atStopS6/integrPaxAlightS1 ==
  ratePax : Inport
  Atomic Subsystem1 : Subsystem  TreatAsAtomicUnit=on
  Round1 : Rounding  Operator=round
  T2E1 : TimedToEventSignal
  accPax : Outport
  wires:
  Round1/1 -> T2E1/1
  T2E1/1 -> Atomic Subsystem1/1(In1)
  ratePax/1 -> Round1/1
  Atomic Subsystem1/1(Out1) -> accPax/1

== system simRouteA_v4_11/atStopS6/integrPaxArrS1 ==
  ratePax : Inport
  Atomic Subsystem1 : Subsystem  TreatAsAtomicUnit=on
  Round1 : Rounding  Operator=round
  T2E1 : TimedToEventSignal
  accPax : Outport
  wires:
  Round1/1 -> T2E1/1
  T2E1/1 -> Atomic Subsystem1/1(In1)
  ratePax/1 -> Round1/1
  Atomic Subsystem1/1(Out1) -> accPax/1

== system simRouteA_v4_11/atStopS7/busDwellThisStop ==
  dwellTime : Inport
  Clock2 : Clock
  DummyServer : SingleServer  ServiceTime=0
  FIFO Queue3 : FIFOQueue
  Get Attribute5 : GetAttribute  AttributeName=dwellTime|tStartSrvPax  AttributeMissing=Error|Error  AttributeDefaultValue=1|1  AttributeTreatAsVector=1|1  AttributeSendTiming=After entity departure|After entity departure  EvaluatedDefaultAttributeValue={ []; []}
      settings: OutputPortMap=o1,o2
  Infinite Server : InfiniteServer  ServiceTimeFrom=Signal port t
  Set Attribute3 : SetAttribute  AttributeName=dwellTime|tStartSrvPax  AttributeFrom=Signal port|Signal port  AttributeValue=1|1  AttributeTreatAsVector=1|1  EvaluatedAttributeValue={ []; [] }
      settings: InputPortMap=u0,u1
  Subsystem2 : Subsystem  TreatAsAtomicUnit=on
  T2E4 : TimedToEventSignal
  busWaitAtStop : SingleServer  Commented=on  ServiceTimeFrom=Signal port t
  busesQueueAtStop : FIFOQueue
  getIDBusLeave : GetAttribute  AttributeName=ID  EvaluatedDefaultAttributeValue={ []}
      settings: OutputPortMap=o1
  busOut : PMIOPort  Port=1  Side=Right
  busIn : PMIOPort  Port=2  Side=Left
  idBusLeave : Outport
  wires:
  getIDBusLeave/1 -> idBusLeave/1
  dwellTime/1 -> Set Attribute3/1
  Clock2/1 -> T2E4/1
  T2E4/1 -> Set Attribute3/2
  Get Attribute5/2 -> Subsystem2/2(tStartSrvPax)
  Get Attribute5/1 -> Subsystem2/1(dwellTime)
  Subsystem2/1(dwellTimeNew) -> Infinite Server/1
  connections:
  busIn/RConn1 -- busesQueueAtStop/LConn1
  getIDBusLeave/RConn1 -- busOut/RConn1
  busesQueueAtStop/RConn1 -- Set Attribute3/LConn1
  Infinite Server/RConn1 -- getIDBusLeave/LConn1
  Set Attribute3/RConn1 -- FIFO Queue3/LConn1
  FIFO Queue3/RConn1 -- Get Attribute5/LConn1
  Get Attribute5/RConn1 -- DummyServer/LConn1
  Infinite Server/LConn1 -- DummyServer/RConn1

== system simRouteA_v4_11/atStopS7/calcPaxActivThisStop ==
  Atomic Subsystem : Subsystem  TreatAsAtomicUnit=on
  Event Filter{,1..4} (5 alike) : EventFilter  ExecuteSubsystem=Upon sample time hit  SignalEdgeType=Rising
  FIFO Queue9 : FIFOQueue
  Get attrib S1 : GetAttribute  AttributeName=vacancy|paxBoard|paxRemain|paxWait|intgPaxArr|intgPaxAlight  AttributeMissing=Error|Error|Error|Error|Error|Error  AttributeDefaultValue=1|1|1|1|1|1  AttributeTreatAsVector=1|1|1|1|1|1  AttributeSendTiming=After entity departure|After entity departure|After entity departure|After entity departure|After entity departure|After entity departure  EvaluatedDefaultAttributeValue={ []; []; []; []; []; []}
      settings: OutputPortMap=o1,o2,o3,o4,o5,o6
  Get init attrib S1 : GetAttribute  AttributeName=maxCap|vacancy|paxAlight|paxArr|sec2Brd|ID  AttributeMissing=Error|Error|Error|Error|Error|Error  AttributeDefaultValue=1|1|1|1|1|1  AttributeTreatAsVector=1|1|1|1|1|1  AttributeSendTiming=After entity departure|After entity departure|After entity departure|After entity departure|After entity departure|After entity departure  EvaluatedDefaultAttributeValue={ []; []; []; []; []; []}
      settings: OutputPortMap=o1,o2,o3,o4,o5,o6
  Set attribS1 : SetAttribute  AttributeName=vacancy|paxBoard|paxRemain|paxWait|intgPaxArr|intgPaxAlight  AttributeFrom=Signal port|Signal port|Signal port|Signal port|Signal port|Signal port  AttributeValue=1|1|1|1|1|1  AttributeTreatAsVector=1|1|1|1|1|1  EvaluatedAttributeValue={ []; []; []; []; []; [] }
      settings: InputPortMap=u0,u1,u2,u3,u4,u5
  calcPaxAlightS1 : Subsystem  TreatAsAtomicUnit=on
  calcPaxArrS1 : Subsystem  TreatAsAtomicUnit=on
  busEntityOut : PMIOPort  Port=1  Side=Right
  busEntityIn : PMIOPort  Port=2  Side=Left
  vacanIn : Outport
  paxAlight : Outport  Port=2
  paxArr : Outport  Port=3
  busID : Outport  Port=4
  newVacan : Outport  Port=5
  paxBoard : Outport  Port=6
  paxRemain : Outport  Port=7
  paxWait : Outport  Port=8
  intgPaxArr : Outport  Port=9
  intgPaxAlight : Outport  Port=10
  dwellTime : Outport  Port=11
  wires:
  Event Filter3/1 -> calcPaxArrS1/1(integrPax)
  Event Filter2/1 -> calcPaxAlightS1/1(integrPax)
  Get init attrib S1/6 -> busID/1
  Get init attrib S1/2 -> vacanIn/1, Event Filter1/1
  Get attrib S1/2 -> paxBoard/1
  Atomic Subsystem/1(newVacancy) -> Set attribS1/1
  Get attrib S1/1 -> newVacan/1
  Get attrib S1/3 -> paxRemain/1
  Get attrib S1/4 -> paxWait/1
  Event Filter/1 -> Atomic Subsystem/1(maxCap)
  Get init attrib S1/5 -> Event Filter4/1
  Atomic Subsystem/5(dwellTime) -> dwellTime/1
  Event Filter1/1 -> Atomic Subsystem/2(vacancy)
  Get init attrib S1/1 -> Event Filter/1
  Event Filter4/1 -> Atomic Subsystem/5(sec2Brd)
  Atomic Subsystem/2(paxBoard) -> Set attribS1/2
  Atomic Subsystem/3(paxRemain) -> Set attribS1/3
  Atomic Subsystem/4(paxWait) -> Set attribS1/4
  Get init attrib S1/4 -> Event Filter3/1
  Get init attrib S1/3 -> Event Filter2/1
  calcPaxAlightS1/1(truPax) -> Atomic Subsystem/3(paxAlight)
  calcPaxArrS1/1(truPax) -> Atomic Subsystem/4(paxArr), paxArr/1
  calcPaxArrS1/2(intgPax) -> Set attribS1/5
  calcPaxAlightS1/2(intgPax) -> Set attribS1/6
  Get attrib S1/5 -> intgPaxArr/1
  Get attrib S1/6 -> intgPaxAlight/1
  Atomic Subsystem/6(corrPaxAlight) -> paxAlight/1
  connections:
  busEntityIn/RConn1 -- Get init attrib S1/LConn1
  FIFO Queue9/LConn1 -- Get init attrib S1/RConn1
  Set attribS1/RConn1 -- Get attrib S1/LConn1
  Get attrib S1/RConn1 -- busEntityOut/RConn1
  FIFO Queue9/RConn1 -- Set attribS1/LConn1

== system simRouteA_v4_11/atStopS7/integrPaxAlightS1 ==
  ratePax : Inport
  Atomic Subsystem1 : Subsystem  TreatAsAtomicUnit=on
  Round1 : Rounding  Operator=round
  T2E1 : TimedToEventSignal
  accPax : Outport
  wires:
  Round1/1 -> T2E1/1
  T2E1/1 -> Atomic Subsystem1/1(In1)
  ratePax/1 -> Round1/1
  Atomic Subsystem1/1(Out1) -> accPax/1

== system simRouteA_v4_11/atStopS7/integrPaxArrS1 ==
  ratePax : Inport
  Atomic Subsystem1 : Subsystem  TreatAsAtomicUnit=on
  Round1 : Rounding  Operator=round
  T2E1 : TimedToEventSignal
  accPax : Outport
  wires:
  Round1/1 -> T2E1/1
  T2E1/1 -> Atomic Subsystem1/1(In1)
  ratePax/1 -> Round1/1
  Atomic Subsystem1/1(Out1) -> accPax/1

== system simRouteA_v4_11/atStopS8/busDwellThisStop ==
  dwellTime : Inport
  Clock2 : Clock
  DummyServer : SingleServer  ServiceTime=0
  FIFO Queue3 : FIFOQueue
  Get Attribute5 : GetAttribute  AttributeName=dwellTime|tStartSrvPax  AttributeMissing=Error|Error  AttributeDefaultValue=1|1  AttributeTreatAsVector=1|1  AttributeSendTiming=After entity departure|After entity departure  EvaluatedDefaultAttributeValue={ []; []}
      settings: OutputPortMap=o1,o2
  Infinite Server : InfiniteServer  ServiceTimeFrom=Signal port t
  Set Attribute3 : SetAttribute  AttributeName=dwellTime|tStartSrvPax  AttributeFrom=Signal port|Signal port  AttributeValue=1|1  AttributeTreatAsVector=1|1  EvaluatedAttributeValue={ []; [] }
      settings: InputPortMap=u0,u1
  Subsystem2 : Subsystem  TreatAsAtomicUnit=on
  T2E4 : TimedToEventSignal
  busWaitAtStop : SingleServer  Commented=on  ServiceTimeFrom=Signal port t
  busesQueueAtStop : FIFOQueue
  getIDBusLeave : GetAttribute  AttributeName=ID  EvaluatedDefaultAttributeValue={ []}
      settings: OutputPortMap=o1
  busOut : PMIOPort  Port=1  Side=Right
  busIn : PMIOPort  Port=2  Side=Left
  idBusLeave : Outport
  wires:
  getIDBusLeave/1 -> idBusLeave/1
  dwellTime/1 -> Set Attribute3/1
  Clock2/1 -> T2E4/1
  T2E4/1 -> Set Attribute3/2
  Get Attribute5/2 -> Subsystem2/2(tStartSrvPax)
  Get Attribute5/1 -> Subsystem2/1(dwellTime)
  Subsystem2/1(dwellTimeNew) -> Infinite Server/1
  connections:
  busIn/RConn1 -- busesQueueAtStop/LConn1
  getIDBusLeave/RConn1 -- busOut/RConn1
  busesQueueAtStop/RConn1 -- Set Attribute3/LConn1
  Infinite Server/RConn1 -- getIDBusLeave/LConn1
  Set Attribute3/RConn1 -- FIFO Queue3/LConn1
  FIFO Queue3/RConn1 -- Get Attribute5/LConn1
  Get Attribute5/RConn1 -- DummyServer/LConn1
  Infinite Server/LConn1 -- DummyServer/RConn1

== system simRouteA_v4_11/atStopS8/calcPaxActivThisStop ==
  Atomic Subsystem : Subsystem  TreatAsAtomicUnit=on
  Event Filter{,1..4} (5 alike) : EventFilter  ExecuteSubsystem=Upon sample time hit  SignalEdgeType=Rising
  FIFO Queue9 : FIFOQueue
  Get attrib S1 : GetAttribute  AttributeName=vacancy|paxBoard|paxRemain|paxWait|intgPaxArr|intgPaxAlight  AttributeMissing=Error|Error|Error|Error|Error|Error  AttributeDefaultValue=1|1|1|1|1|1  AttributeTreatAsVector=1|1|1|1|1|1  AttributeSendTiming=After entity departure|After entity departure|After entity departure|After entity departure|After entity departure|After entity departure  EvaluatedDefaultAttributeValue={ []; []; []; []; []; []}
      settings: OutputPortMap=o1,o2,o3,o4,o5,o6
  Get init attrib S1 : GetAttribute  AttributeName=maxCap|vacancy|paxAlight|paxArr|sec2Brd|ID  AttributeMissing=Error|Error|Error|Error|Error|Error  AttributeDefaultValue=1|1|1|1|1|1  AttributeTreatAsVector=1|1|1|1|1|1  AttributeSendTiming=After entity departure|After entity departure|After entity departure|After entity departure|After entity departure|After entity departure  EvaluatedDefaultAttributeValue={ []; []; []; []; []; []}
      settings: OutputPortMap=o1,o2,o3,o4,o5,o6
  Set attribS1 : SetAttribute  AttributeName=vacancy|paxBoard|paxRemain|paxWait|intgPaxArr|intgPaxAlight  AttributeFrom=Signal port|Signal port|Signal port|Signal port|Signal port|Signal port  AttributeValue=1|1|1|1|1|1  AttributeTreatAsVector=1|1|1|1|1|1  EvaluatedAttributeValue={ []; []; []; []; []; [] }
      settings: InputPortMap=u0,u1,u2,u3,u4,u5
  calcPaxAlightS1 : Subsystem  TreatAsAtomicUnit=on
  calcPaxArrS1 : Subsystem  TreatAsAtomicUnit=on
  busEntityOut : PMIOPort  Port=1  Side=Right
  busEntityIn : PMIOPort  Port=2  Side=Left
  vacanIn : Outport
  paxAlight : Outport  Port=2
  paxArr : Outport  Port=3
  busID : Outport  Port=4
  newVacan : Outport  Port=5
  paxBoard : Outport  Port=6
  paxRemain : Outport  Port=7
  paxWait : Outport  Port=8
  intgPaxArr : Outport  Port=9
  intgPaxAlight : Outport  Port=10
  dwellTime : Outport  Port=11
  wires:
  Event Filter3/1 -> calcPaxArrS1/1(integrPax)
  Event Filter2/1 -> calcPaxAlightS1/1(integrPax)
  Get init attrib S1/6 -> busID/1
  Get init attrib S1/2 -> vacanIn/1, Event Filter1/1
  Get attrib S1/2 -> paxBoard/1
  Atomic Subsystem/1(newVacancy) -> Set attribS1/1
  Get attrib S1/1 -> newVacan/1
  Get attrib S1/3 -> paxRemain/1
  Get attrib S1/4 -> paxWait/1
  Event Filter/1 -> Atomic Subsystem/1(maxCap)
  Get init attrib S1/5 -> Event Filter4/1
  Atomic Subsystem/5(dwellTime) -> dwellTime/1
  Event Filter1/1 -> Atomic Subsystem/2(vacancy)
  Get init attrib S1/1 -> Event Filter/1
  Event Filter4/1 -> Atomic Subsystem/5(sec2Brd)
  Atomic Subsystem/2(paxBoard) -> Set attribS1/2
  Atomic Subsystem/3(paxRemain) -> Set attribS1/3
  Atomic Subsystem/4(paxWait) -> Set attribS1/4
  Get init attrib S1/4 -> Event Filter3/1
  Get init attrib S1/3 -> Event Filter2/1
  calcPaxAlightS1/1(truPax) -> Atomic Subsystem/3(paxAlight)
  calcPaxArrS1/1(truPax) -> Atomic Subsystem/4(paxArr), paxArr/1
  calcPaxArrS1/2(intgPax) -> Set attribS1/5
  calcPaxAlightS1/2(intgPax) -> Set attribS1/6
  Get attrib S1/5 -> intgPaxArr/1
  Get attrib S1/6 -> intgPaxAlight/1
  Atomic Subsystem/6(corrPaxAlight) -> paxAlight/1
  connections:
  busEntityIn/RConn1 -- Get init attrib S1/LConn1
  FIFO Queue9/LConn1 -- Get init attrib S1/RConn1
  Set attribS1/RConn1 -- Get attrib S1/LConn1
  Get attrib S1/RConn1 -- busEntityOut/RConn1
  FIFO Queue9/RConn1 -- Set attribS1/LConn1

== system simRouteA_v4_11/atStopS8/integrPaxAlightS1 ==
  ratePax : Inport
  Atomic Subsystem1 : Subsystem  TreatAsAtomicUnit=on
  Round1 : Rounding  Operator=round
  T2E1 : TimedToEventSignal
  accPax : Outport
  wires:
  Round1/1 -> T2E1/1
  T2E1/1 -> Atomic Subsystem1/1(In1)
  ratePax/1 -> Round1/1
  Atomic Subsystem1/1(Out1) -> accPax/1

== system simRouteA_v4_11/atStopS8/integrPaxArrS1 ==
  ratePax : Inport
  Atomic Subsystem1 : Subsystem  TreatAsAtomicUnit=on
  Round1 : Rounding  Operator=round
  T2E1 : TimedToEventSignal
  accPax : Outport
  wires:
  Round1/1 -> T2E1/1
  T2E1/1 -> Atomic Subsystem1/1(In1)
  ratePax/1 -> Round1/1
  Atomic Subsystem1/1(Out1) -> accPax/1

== system simRouteA_v4_11/atStopS9/busDwellThisStop ==
  dwellTime : Inport
  Clock2 : Clock
  DummyServer : SingleServer  ServiceTime=0
  FIFO Queue3 : FIFOQueue
  Get Attribute5 : GetAttribute  AttributeName=dwellTime|tStartSrvPax  AttributeMissing=Error|Error  AttributeDefaultValue=1|1  AttributeTreatAsVector=1|1  AttributeSendTiming=After entity departure|After entity departure  EvaluatedDefaultAttributeValue={ []; []}
      settings: OutputPortMap=o1,o2
  Infinite Server : InfiniteServer  ServiceTimeFrom=Signal port t
  Set Attribute3 : SetAttribute  AttributeName=dwellTime|tStartSrvPax  AttributeFrom=Signal port|Signal port  AttributeValue=1|1  AttributeTreatAsVector=1|1  EvaluatedAttributeValue={ []; [] }
      settings: InputPortMap=u0,u1
  Subsystem2 : Subsystem  TreatAsAtomicUnit=on
  T2E4 : TimedToEventSignal
  busWaitAtStop : SingleServer  Commented=on  ServiceTimeFrom=Signal port t
  busesQueueAtStop : FIFOQueue
  getIDBusLeave : GetAttribute  AttributeName=ID  EvaluatedDefaultAttributeValue={ []}
      settings: OutputPortMap=o1
  busOut : PMIOPort  Port=1  Side=Right
  busIn : PMIOPort  Port=2  Side=Left
  idBusLeave : Outport
  wires:
  getIDBusLeave/1 -> idBusLeave/1
  dwellTime/1 -> Set Attribute3/1
  Clock2/1 -> T2E4/1
  T2E4/1 -> Set Attribute3/2
  Get Attribute5/2 -> Subsystem2/2(tStartSrvPax)
  Get Attribute5/1 -> Subsystem2/1(dwellTime)
  Subsystem2/1(dwellTimeNew) -> Infinite Server/1
  connections:
  busIn/RConn1 -- busesQueueAtStop/LConn1
  getIDBusLeave/RConn1 -- busOut/RConn1
  busesQueueAtStop/RConn1 -- Set Attribute3/LConn1
  Infinite Server/RConn1 -- getIDBusLeave/LConn1
  Set Attribute3/RConn1 -- FIFO Queue3/LConn1
  FIFO Queue3/RConn1 -- Get Attribute5/LConn1
  Get Attribute5/RConn1 -- DummyServer/LConn1
  Infinite Server/LConn1 -- DummyServer/RConn1

== system simRouteA_v4_11/atStopS9/calcPaxActivThisStop ==
  Atomic Subsystem : Subsystem  TreatAsAtomicUnit=on
  Event Filter{,1..4} (5 alike) : EventFilter  ExecuteSubsystem=Upon sample time hit  SignalEdgeType=Rising
  FIFO Queue9 : FIFOQueue
  Get attrib S1 : GetAttribute  AttributeName=vacancy|paxBoard|paxRemain|paxWait|intgPaxArr|intgPaxAlight  AttributeMissing=Error|Error|Error|Error|Error|Error  AttributeDefaultValue=1|1|1|1|1|1  AttributeTreatAsVector=1|1|1|1|1|1  AttributeSendTiming=After entity departure|After entity departure|After entity departure|After entity departure|After entity departure|After entity departure  EvaluatedDefaultAttributeValue={ []; []; []; []; []; []}
      settings: OutputPortMap=o1,o2,o3,o4,o5,o6
  Get init attrib S1 : GetAttribute  AttributeName=maxCap|vacancy|paxAlight|paxArr|sec2Brd|ID  AttributeMissing=Error|Error|Error|Error|Error|Error  AttributeDefaultValue=1|1|1|1|1|1  AttributeTreatAsVector=1|1|1|1|1|1  AttributeSendTiming=After entity departure|After entity departure|After entity departure|After entity departure|After entity departure|After entity departure  EvaluatedDefaultAttributeValue={ []; []; []; []; []; []}
      settings: OutputPortMap=o1,o2,o3,o4,o5,o6
  Set attribS1 : SetAttribute  AttributeName=vacancy|paxBoard|paxRemain|paxWait|intgPaxArr|intgPaxAlight  AttributeFrom=Signal port|Signal port|Signal port|Signal port|Signal port|Signal port  AttributeValue=1|1|1|1|1|1  AttributeTreatAsVector=1|1|1|1|1|1  EvaluatedAttributeValue={ []; []; []; []; []; [] }
      settings: InputPortMap=u0,u1,u2,u3,u4,u5
  calcPaxAlightS1 : Subsystem  TreatAsAtomicUnit=on
  calcPaxArrS1 : Subsystem  TreatAsAtomicUnit=on
  busEntityOut : PMIOPort  Port=1  Side=Right
  busEntityIn : PMIOPort  Port=2  Side=Left
  vacanIn : Outport
  paxAlight : Outport  Port=2
  paxArr : Outport  Port=3
  busID : Outport  Port=4
  newVacan : Outport  Port=5
  paxBoard : Outport  Port=6
  paxRemain : Outport  Port=7
  paxWait : Outport  Port=8
  intgPaxArr : Outport  Port=9
  intgPaxAlight : Outport  Port=10
  dwellTime : Outport  Port=11
  wires:
  Event Filter3/1 -> calcPaxArrS1/1(integrPax)
  Event Filter2/1 -> calcPaxAlightS1/1(integrPax)
  Get init attrib S1/6 -> busID/1
  Get init attrib S1/2 -> vacanIn/1, Event Filter1/1
  Get attrib S1/2 -> paxBoard/1
  Atomic Subsystem/1(newVacancy) -> Set attribS1/1
  Get attrib S1/1 -> newVacan/1
  Get attrib S1/3 -> paxRemain/1
  Get attrib S1/4 -> paxWait/1
  Event Filter/1 -> Atomic Subsystem/1(maxCap)
  Get init attrib S1/5 -> Event Filter4/1
  Atomic Subsystem/5(dwellTime) -> dwellTime/1
  Event Filter1/1 -> Atomic Subsystem/2(vacancy)
  Get init attrib S1/1 -> Event Filter/1
  Event Filter4/1 -> Atomic Subsystem/5(sec2Brd)
  Atomic Subsystem/2(paxBoard) -> Set attribS1/2
  Atomic Subsystem/3(paxRemain) -> Set attribS1/3
  Atomic Subsystem/4(paxWait) -> Set attribS1/4
  Get init attrib S1/4 -> Event Filter3/1
  Get init attrib S1/3 -> Event Filter2/1
  calcPaxAlightS1/1(truPax) -> Atomic Subsystem/3(paxAlight)
  calcPaxArrS1/1(truPax) -> Atomic Subsystem/4(paxArr), paxArr/1
  calcPaxArrS1/2(intgPax) -> Set attribS1/5
  calcPaxAlightS1/2(intgPax) -> Set attribS1/6
  Get attrib S1/5 -> intgPaxArr/1
  Get attrib S1/6 -> intgPaxAlight/1
  Atomic Subsystem/6(corrPaxAlight) -> paxAlight/1
  connections:
  busEntityIn/RConn1 -- Get init attrib S1/LConn1
  FIFO Queue9/LConn1 -- Get init attrib S1/RConn1
  Set attribS1/RConn1 -- Get attrib S1/LConn1
  Get attrib S1/RConn1 -- busEntityOut/RConn1
  FIFO Queue9/RConn1 -- Set attribS1/LConn1

== system simRouteA_v4_11/atStopS9/integrPaxAlightS1 ==
  ratePax : Inport
  Atomic Subsystem1 : Subsystem  TreatAsAtomicUnit=on
  Round1 : Rounding  Operator=round
  T2E1 : TimedToEventSignal
  accPax : Outport
  wires:
  Round1/1 -> T2E1/1
  T2E1/1 -> Atomic Subsystem1/1(In1)
  ratePax/1 -> Round1/1
  Atomic Subsystem1/1(Out1) -> accPax/1

== system simRouteA_v4_11/atStopS9/integrPaxArrS1 ==
  ratePax : Inport
  Atomic Subsystem1 : Subsystem  TreatAsAtomicUnit=on
  Round1 : Rounding  Operator=round
  T2E1 : TimedToEventSignal
  accPax : Outport
  wires:
  Round1/1 -> T2E1/1
  T2E1/1 -> Atomic Subsystem1/1(In1)
  ratePax/1 -> Round1/1
  Atomic Subsystem1/1(Out1) -> accPax/1

== system simRouteA_v4_11/chkSchedTimeNormalBusAtCP2/Subsystem2 ==
  ID : Inport
  tTable : Inport  Port=2
  Constant12 : Constant  Value=10000
  Constant13 : Constant
  Direct Lookup Table (n-D)1 : LookupNDDirect  TableIsInput=on
  Divide1 : Product  Inputs=/*
  Math Function1 : Math  Operator=mod  SaturateOnIntegerOverflow=on
  Rounding : Rounding  Operator=round
  Rounding1 : Rounding  Operator=round
  Subtract1 : Sum  Inputs=-+
  schedTime : Outport
  wires:
  Rounding1/1 -> Direct Lookup Table (n-D)1/1
  Constant12/1 -> Math Function1/2, Divide1/1
  Constant13/1 -> Subtract1/1
  Divide1/1 -> Rounding/1
  Subtract1/1 -> Direct Lookup Table (n-D)1/2
  Direct Lookup Table (n-D)1/1 -> schedTime/1
  tTable/1 -> Direct Lookup Table (n-D)1/3
  Math Function1/1 -> Rounding1/1
  Rounding/1 -> Subtract1/2
  ID/1 -> Divide1/2, Math Function1/1

== system simRouteA_v4_11/chkSchedTimeNormalBusAtCP2/While Iterator Subsystem ==
  crnBusID : Inport
  timetableAtStart : Inport  Port=2
  crnTimeAtCP : Inport  Port=3
  IC : Inport  Port=4
  Add1 : Sum
  Constant2 : Constant  Value=10000
  Constant4 : Constant
  Direct Lookup Table (n-D)2 : LookupNDDirect  TableIsInput=on
  Divide2 : Product  Inputs=/*
  Math Function1 : Math  Operator=mod  SaturateOnIntegerOverflow=on
  Memory : Memory
  Relational Operator : RelationalOperator  Operator=<=  OutDataTypeStr=boolean
  Rounding2 : Rounding  Operator=round
  Rounding3 : Rounding  Operator=round
  Subtract2 : Sum  Inputs=-+
  Sum : Sum  Inputs=|++
  While Iterator : WhileIterator  ShowIterationPort=on
  nxtDepTimeAtStart : Outport
  nxtBusID : Outport  Port=2
  wires:
  IC/1 -> While Iterator/2
  While Iterator/1 -> Sum/1
  Memory/1 -> Sum/2
  Sum/1 -> Add1/2, Memory/1
  crnBusID/1 -> Add1/1
  Rounding2/1 -> Direct Lookup Table (n-D)2/1
  Divide2/1 -> Rounding3/1
  Add1/1 -> Divide2/2, nxtBusID/1, Math Function1/1
  Math Function1/1 -> Rounding2/1
  Constant2/1 -> Divide2/1, Math Function1/2
  timetableAtStart/1 -> Direct Lookup Table (n-D)2/3
  Rounding3/1 -> Subtract2/2
  Constant4/1 -> Subtract2/1
  Subtract2/1 -> Direct Lookup Table (n-D)2/2
  Direct Lookup Table (n-D)2/1 -> Relational Operator/1, nxtDepTimeAtStart/1
  crnTimeAtCP/1 -> Relational Operator/2
  Relational Operator/1 -> While Iterator/1
